simulink model "ex_lqr_robot_simulink"  (R2022b)
settings: Solver=VariableStepAuto  StartTime=0.0  StopTime=5  RelTol=1e-12
InitFcn:
  | ex_lqr_robot_eqs
values from neighbouring files (symbols this model uses):
  C = [1, 0, 0, 0 ... (first row only)    [ex_lqr.m]    (also in ex_lqr_robot_eqs.m = [1 0 0 0 ; 0 0 1 0]; ex_lqr_robot_linear.m; ex_pi_gain_optimization.m = pid(Kp,Ki))
  K = K1(:,1:4)    [ex_lqr_robot_eqs.m]
  Ki = -K1(:,5:6)    [ex_lqr_robot_eqs.m]    (also in ex_pi_gain_optimization.m = gains(2))
  u0 = [tau10; tau20]    [ex_lqr_robot_eqs.m]
  x0 = [T10; 0; T20; 0]    [ex_lqr_robot_eqs.m]    (also in ex_pi_gain_optimization.m = [KP0;KI0])
settings Model: Creator=Dan  LastModifiedBy=Dan
settings SolverCC: InitialStep=1e-12
settings DataIOCC: SaveFormat=Array

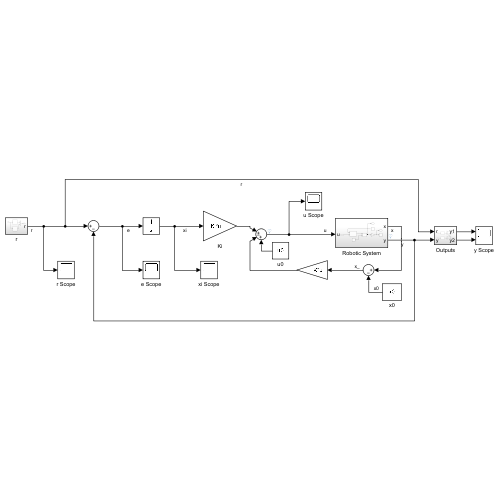
[thumbnail: Simulink's stored preview of the top-level diagram]
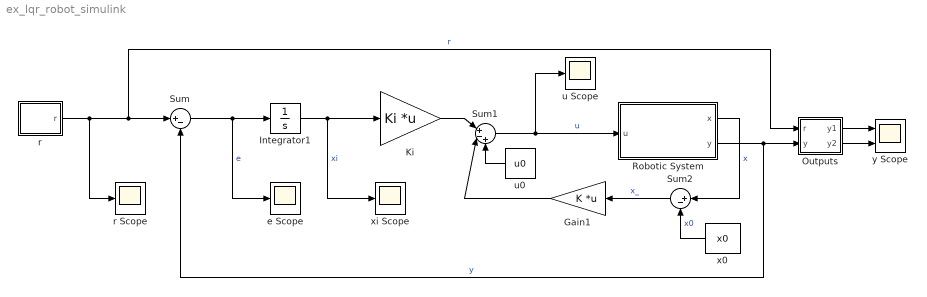
== system ex_lqr_robot_simulink ==
  Gain1 : Gain  Gain=K  Multiplication=Matrix(K*u)
  Integrator1 : Integrator
  Ki : Gain  Gain=Ki  Multiplication=Matrix(K*u)
  Outputs : Subsystem
  Robotic System : Subsystem
  Sum : Sum  Inputs=|+-
  Sum1 : Sum  Inputs=|+-+
  Sum2 : Sum  Inputs=|+-
  e Scope : Scope
  r : Subsystem
  r Scope : Scope
  u Scope : Scope
  u0 : Constant  Value=u0  VectorParams1D=off
  x0 : Constant  Value=x0  VectorParams1D=off
  xi Scope : Scope
  y Scope : Scope  NumInputPorts=2
  wires:
  Sum1/1 -> u Scope/1, Robotic System/1(u)  "u"
  u0/1 -> Sum1/3
  Robotic System/1(x) -> Sum2/1  "x"
  Robotic System/2(y) -> Outputs/2(y), Sum/2  "y"
  Gain1/1 -> Sum1/2
  Sum/1 -> Integrator1/1, e Scope/1  "e"
  Sum2/1 -> Gain1/1  "x_"
  x0/1 -> Sum2/2  "x0"
  Integrator1/1 -> Ki/1, xi Scope/1  "xi"
  Ki/1 -> Sum1/1
  Outputs/1(y1) -> y Scope/1
  Outputs/2(y2) -> y Scope/2
  r/1(r) -> r Scope/1, Sum/1, Outputs/1(r)  "r"

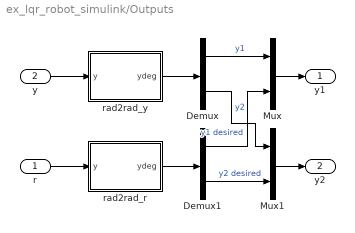
== system ex_lqr_robot_simulink/Outputs ==
  r : Inport
  y : Inport  Port=2
  Demux : Demux  Outputs=2
  Demux1 : Demux  Outputs=2
  Mux : Mux  Inputs=2
  Mux1 : Mux  Inputs=2
  rad2rad_r : MATLAB Function  TreatAsAtomicUnit=on
  rad2rad_y : MATLAB Function  TreatAsAtomicUnit=on
  y1 : Outport
  y2 : Outport  Port=2
  wires:
  Demux1/1 -> Mux/2  "y1 desired"
  Demux/2 -> Mux1/1  "y2"
  r/1 -> rad2rad_r/1(y)
  y/1 -> rad2rad_y/1(y)
  rad2rad_y/1(ydeg) -> Demux/1
  rad2rad_r/1(ydeg) -> Demux1/1
  Demux/1 -> Mux/1  "y1"
  Demux1/2 -> Mux1/2  "y2 desired"
  Mux/1 -> y1/1
  Mux1/1 -> y2/1

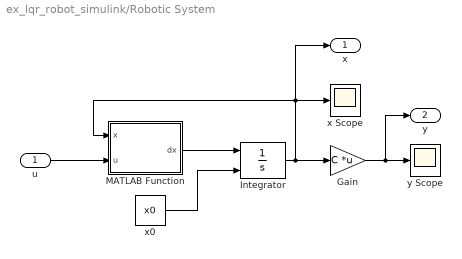
== system ex_lqr_robot_simulink/Robotic System ==
  u : Inport
  Gain : Gain  Gain=C  Multiplication=Matrix(K*u)
  Integrator : Integrator  InitialConditionSource=external
  MATLAB Function : MATLAB Function  TreatAsAtomicUnit=on
  x Scope : Scope
  x0 : Constant  Value=x0  VectorParams1D=off
  y Scope : Scope
  x : Outport
  y : Outport  Port=2
  wires:
  x0/1 -> Integrator/2
  MATLAB Function/1(dx) -> Integrator/1
  Integrator/1 -> x Scope/1, x/1, MATLAB Function/1(x), Gain/1
  u/1 -> MATLAB Function/2(u)
  Gain/1 -> y Scope/1, y/1

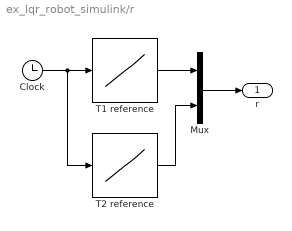
== system ex_lqr_robot_simulink/r ==
  Clock : Clock
  Mux : Mux  Inputs=2
  T1 reference : Lookup_n-D  NumberOfTableDimensions=1  BreakpointsForDimension1=[0 0.1 3]  Table=deg2rad([45 -45 -45])  InterpMethod=Flat  InternalRulePriority=Speed  RndMeth=Simplest
  T2 reference : Lookup_n-D  NumberOfTableDimensions=1  BreakpointsForDimension1=[0 0.1 3]  Table=deg2rad([-30 -30 30])  InterpMethod=Flat  InternalRulePriority=Speed  RndMeth=Simplest
  r : Outport
  wires:
  Mux/1 -> r/1
  T2 reference/1 -> Mux/2
  T1 reference/1 -> Mux/1
  Clock/1 -> T2 reference/1, T1 reference/1

== matlab function ex_lqr_robot_simulink/Outputs/rad2rad_y ==
  data: y input; ydeg output
function ydeg = fcn(y)

ydeg = rad2deg(y);

== matlab function ex_lqr_robot_simulink/Robotic System/MATLAB Function ==
  data: x input; dx output; u input
function dx = fcn(x,u)

% T10 = deg2rad(45);
% DT10 = deg2rad(0);
% T20 = deg2rad(-30);
% DT20 = deg2rad(0);

T10 = x(1);
DT10 = x(2);
T20 = x(3);
DT20 = x(4);

J1 = 0.12;
J2 = 0.15;
g = 9.81;
l1 = 0.6;
l2 = 0.8;
m1 = 3;
m2 = 2.5;

M11 = (1/4*m1+m2)*l1^2 + 1/4*m2*l2^2 + J1 + J2 + m2*l1*l2*cos(T20);
M12 = 1/4*m2*l2^2 + J2 + 1/2*m2*l1*l2*cos(T20);
M22 = 1/4*m2*l2^2 + J2;

M = [M11 M12; M12 M22];

H = inv(M);

H11 = H(1,1);
H12 = H(1,2);
H21 = H(2,1);
H22 = H(2,2);

K1 = -1/2*m2*l1*l2*sin(T20)*DT20*(2*DT10 + DT20);
K2 = 1/2*m2*l1*l2*sin(T20)*DT10^2;

G1 = m1*g*l1/2*cos(T10) + m2*g*(l1*cos(T10) + l2/2*cos(T10+T20));
G2 = m2*g*l2/2*cos(T10+T20);

dx = zeros(4,1);
dx(1) = x(2);
dx(2) = -H11*(K1+G1) - H12*(K2+G2) + [H11 H12]*u;
dx(3) = x(4);
dx(4) = -H21*(K1+G1) - H22*(K2+G2) + [H21 H22]*u;

end

== matlab function ex_lqr_robot_simulink/Outputs/rad2rad_r ==
  data: y input; ydeg output
function ydeg = fcn(y)

ydeg = rad2deg(y);
